simulink model "mult_friction_observer"  (R2021a)
settings: Solver=FixedStepAuto  StartTime=0.0  StopTime=10.0  RelTol=1e-3
model workspace (MAT data in the model file):
  C = [1  0  0  0  0  0  0  0; 0  1  0  0  0  0  0  0; 0  0  1  0  0  0  0  0; 0  0  0  1  0  0  0  0]
  Gamma = [0.005  0  0  0; 0  0.005  0  0; 0  0  0.005  0; 0  0  0  0.005; 0  0  0  0; 0  0  0  0; 0  0  0  0; 0  0  0  0]
  L = [0.86054447364  -0.080292367616  -0.128389264309  0.0921786693579; 0.0643400875833  0.825287721844  0.151017179007  0.010258969185; -0.0245436500305  -0.0437560245931  0.828239855806  -0.0359294386871; -0.0985279277998  0.00654816106119  0.213243264372  0.710326675841; -86.465018388  -7.61905487874  13.7748818427  -3.05301802345; -2.05392908471  -74.8278985038  -8.19625899202  -1.35897353285; 5.97220378745  -11.304802381  -76.7309175474  -0.134671122007; -11.4863013293  -16.7435461743  -5.18969499217  -60.1810056818]
  Phi = [1  0  0  0  -0.0016511627907  0  0  0; 0  1  0  0  0  -0.0016511627907  0  0; 0  0  1  0  0  0  -0.00160888284614  0; 0  0  0  1  0  0  0  -0.00160888284614; 0  0  0  0  1  0  0  0; 0  0  0  0  0  1  0  0; 0  0  0  0  0  0  1  0; 0  0  0  0  0  0  0  1]
  Ts = 0.005
settings Model: OrderedModelArguments=off  Creator=Henrique Mesquita  LastModifiedBy=Henrique Mesquita

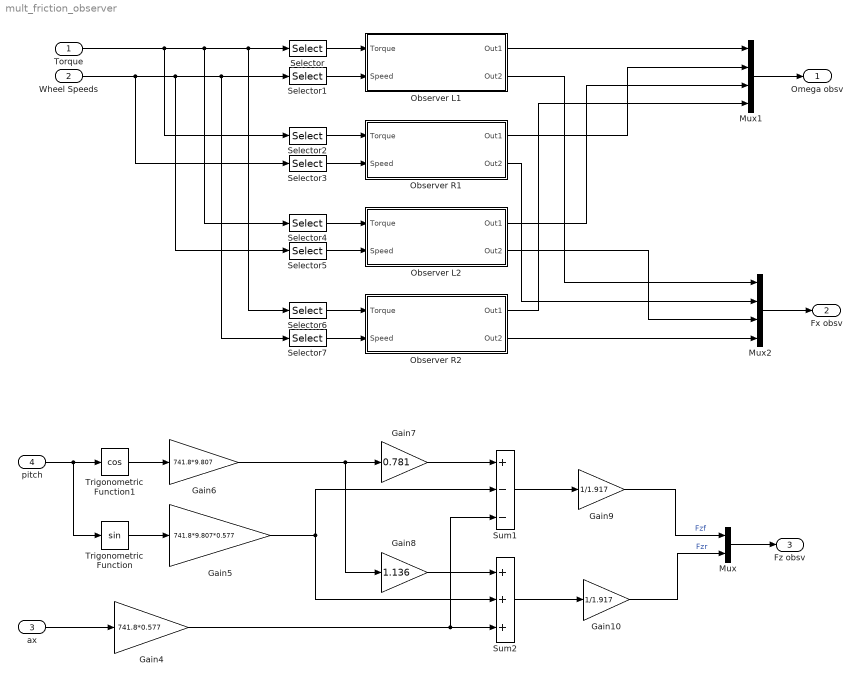
== system mult_friction_observer ==
  Torque : Inport  PortDimensions=4
  Wheel Speeds : Inport  Port=2  PortDimensions=4
  ax : Inport  Port=3
  pitch : Inport  Port=4
  Gain10 : Gain  Gain=1/1.917
  Gain4 : Gain  Gain=741.8*0.577
  Gain5 : Gain  Gain=741.8*9.807*0.577
  Gain6 : Gain  Gain=741.8*9.807
  Gain7 : Gain  Gain=0.781
  Gain8 : Gain  Gain=1.136
  Gain9 : Gain  Gain=1/1.917
  Mux : Mux  Inputs=2
  Mux1 : Mux
  Mux2 : Mux
  Observer L1 : Subsystem
  Observer L2 : Subsystem
  Observer R1 : Subsystem
  Observer R2 : Subsystem
  Selector : Selector  InputPortWidth=4  IndexOptions=Index vector (dialog)  Indices=[1]  OutputSizes=1
  Selector1 : Selector  InputPortWidth=4  IndexOptions=Index vector (dialog)  Indices=[1]  OutputSizes=1
  Selector2 : Selector  InputPortWidth=4  IndexOptions=Index vector (dialog)  Indices=[1]  OutputSizes=1
  Selector3 : Selector  InputPortWidth=4  IndexOptions=Index vector (dialog)  Indices=[2]  OutputSizes=1
  Selector4 : Selector  InputPortWidth=4  IndexOptions=Index vector (dialog)  Indices=[3]  OutputSizes=1
  Selector5 : Selector  InputPortWidth=4  IndexOptions=Index vector (dialog)  Indices=[3]  OutputSizes=1
  Selector6 : Selector  InputPortWidth=4  IndexOptions=Index vector (dialog)  Indices=[4]  OutputSizes=1
  Selector7 : Selector  InputPortWidth=4  IndexOptions=Index vector (dialog)  Indices=[4]  OutputSizes=1
  Sum1 : Sum  Inputs=+--
  Sum2 : Sum  Inputs=+++
  Trigonometric Function : Trigonometry
  Trigonometric Function1 : Trigonometry  Operator=cos
  Omega obsv : Outport
  Fx obsv : Outport  Port=2
  Fz obsv : Outport  Port=3
  wires:
  pitch/1 -> Trigonometric Function/1, Trigonometric Function1/1
  Trigonometric Function/1 -> Gain5/1
  Trigonometric Function1/1 -> Gain6/1
  Gain6/1 -> Gain8/1, Gain7/1
  Gain7/1 -> Sum1/1
  Gain8/1 -> Sum2/1
  Gain5/1 -> Sum2/2, Sum1/2
  ax/1 -> Gain4/1
  Gain4/1 -> Sum1/3, Sum2/3
  Sum1/1 -> Gain9/1
  Sum2/1 -> Gain10/1
  Gain9/1 -> Mux/1  "Fzf"
  Gain10/1 -> Mux/2  "Fzr"
  Mux/1 -> Fz obsv/1
  Wheel Speeds/1 -> Selector3/1, Selector5/1, Selector7/1, Selector1/1
  Torque/1 -> Selector2/1, Selector6/1, Selector/1, Selector4/1
  Selector/1 -> Observer L1/1(Torque)
  Selector1/1 -> Observer L1/2(Speed)
  Selector2/1 -> Observer R1/1(Torque)
  Selector3/1 -> Observer R1/2(Speed)
  Selector4/1 -> Observer L2/1(Torque)
  Selector5/1 -> Observer L2/2(Speed)
  Selector6/1 -> Observer R2/1(Torque)
  Selector7/1 -> Observer R2/2(Speed)
  Observer L1/1(Out1) -> Mux1/1
  Observer R1/1(Out1) -> Mux1/2
  Observer L2/1(Out1) -> Mux1/3
  Observer R2/1(Out1) -> Mux1/4
  Observer L1/2(Out2) -> Mux2/1
  Observer R1/2(Out2) -> Mux2/2
  Observer L2/2(Out2) -> Mux2/3
  Observer R2/2(Out2) -> Mux2/4
  Mux2/1 -> Fx obsv/1
  Mux1/1 -> Omega obsv/1

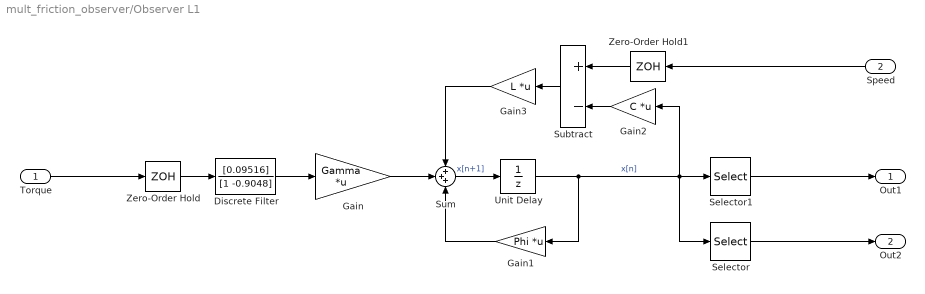
== system mult_friction_observer/Observer L1 ==
  Torque : Inport
  Speed : Inport  Port=2
  Discrete Filter : DiscreteFilter  Numerator=[0.09516]  Denominator=[1 -0.9048]
  Gain : Gain  Gain=Gamma  Multiplication=Matrix(K*u)
  Gain1 : Gain  Gain=Phi  Multiplication=Matrix(K*u)
  Gain2 : Gain  Gain=C  Multiplication=Matrix(K*u)
  Gain3 : Gain  Gain=L  Multiplication=Matrix(K*u)
  Selector : Selector  InputPortWidth=8  IndexOptions=Index vector (dialog)  Indices=[5 6 7 8]  OutputSizes=1
  Selector1 : Selector  InputPortWidth=8  IndexOptions=Index vector (dialog)  Indices=[1 2 3 4]  OutputSizes=1
  Subtract : Sum  Inputs=+-
  Sum : Sum  Inputs=+++
  Unit Delay : UnitDelay  SampleTime=Ts  HasFrameUpgradeWarning=on
  Zero-Order Hold : ZeroOrderHold  SampleTime=Ts
  Zero-Order Hold1 : ZeroOrderHold  SampleTime=Ts
  Out1 : Outport
  Out2 : Outport  Port=2
  wires:
  Sum/1 -> Unit Delay/1  "x[n+1]"
  Unit Delay/1 -> Selector1/1, Selector/1, Gain2/1, Gain1/1  "x[n]"
  Gain3/1 -> Sum/1
  Zero-Order Hold/1 -> Discrete Filter/1
  Subtract/1 -> Gain3/1
  Gain2/1 -> Subtract/2
  Gain1/1 -> Sum/3
  Gain/1 -> Sum/2
  Zero-Order Hold1/1 -> Subtract/1
  Discrete Filter/1 -> Gain/1
  Selector/1 -> Out2/1
  Torque/1 -> Zero-Order Hold/1
  Speed/1 -> Zero-Order Hold1/1
  Selector1/1 -> Out1/1

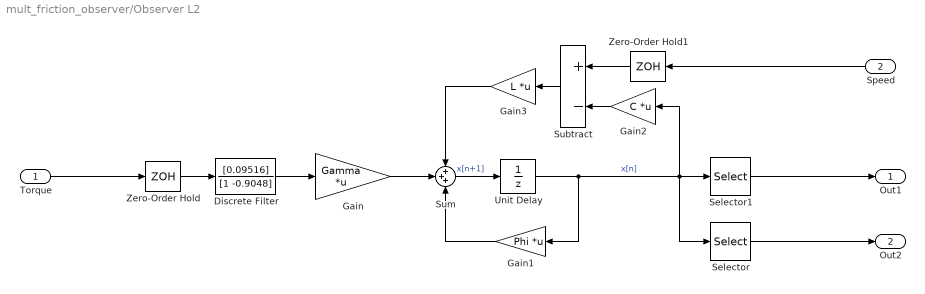
== system mult_friction_observer/Observer L2 ==
  Torque : Inport
  Speed : Inport  Port=2
  Discrete Filter : DiscreteFilter  Numerator=[0.09516]  Denominator=[1 -0.9048]
  Gain : Gain  Gain=Gamma  Multiplication=Matrix(K*u)
  Gain1 : Gain  Gain=Phi  Multiplication=Matrix(K*u)
  Gain2 : Gain  Gain=C  Multiplication=Matrix(K*u)
  Gain3 : Gain  Gain=L  Multiplication=Matrix(K*u)
  Selector : Selector  InputPortWidth=8  IndexOptions=Index vector (dialog)  Indices=[5 6 7 8]  OutputSizes=1
  Selector1 : Selector  InputPortWidth=8  IndexOptions=Index vector (dialog)  Indices=[1 2 3 4]  OutputSizes=1
  Subtract : Sum  Inputs=+-
  Sum : Sum  Inputs=+++
  Unit Delay : UnitDelay  SampleTime=Ts  HasFrameUpgradeWarning=on
  Zero-Order Hold : ZeroOrderHold  SampleTime=Ts
  Zero-Order Hold1 : ZeroOrderHold  SampleTime=Ts
  Out1 : Outport
  Out2 : Outport  Port=2
  wires:
  Sum/1 -> Unit Delay/1  "x[n+1]"
  Unit Delay/1 -> Selector1/1, Selector/1, Gain2/1, Gain1/1  "x[n]"
  Gain3/1 -> Sum/1
  Zero-Order Hold/1 -> Discrete Filter/1
  Subtract/1 -> Gain3/1
  Gain2/1 -> Subtract/2
  Gain1/1 -> Sum/3
  Gain/1 -> Sum/2
  Zero-Order Hold1/1 -> Subtract/1
  Discrete Filter/1 -> Gain/1
  Selector/1 -> Out2/1
  Torque/1 -> Zero-Order Hold/1
  Speed/1 -> Zero-Order Hold1/1
  Selector1/1 -> Out1/1

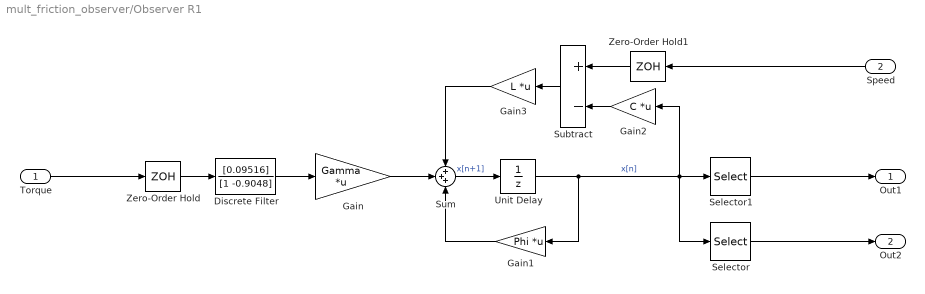
== system mult_friction_observer/Observer R1 ==
  Torque : Inport
  Speed : Inport  Port=2
  Discrete Filter : DiscreteFilter  Numerator=[0.09516]  Denominator=[1 -0.9048]
  Gain : Gain  Gain=Gamma  Multiplication=Matrix(K*u)
  Gain1 : Gain  Gain=Phi  Multiplication=Matrix(K*u)
  Gain2 : Gain  Gain=C  Multiplication=Matrix(K*u)
  Gain3 : Gain  Gain=L  Multiplication=Matrix(K*u)
  Selector : Selector  InputPortWidth=8  IndexOptions=Index vector (dialog)  Indices=[5 6 7 8]  OutputSizes=1
  Selector1 : Selector  InputPortWidth=8  IndexOptions=Index vector (dialog)  Indices=[1 2 3 4]  OutputSizes=1
  Subtract : Sum  Inputs=+-
  Sum : Sum  Inputs=+++
  Unit Delay : UnitDelay  SampleTime=Ts  HasFrameUpgradeWarning=on
  Zero-Order Hold : ZeroOrderHold  SampleTime=Ts
  Zero-Order Hold1 : ZeroOrderHold  SampleTime=Ts
  Out1 : Outport
  Out2 : Outport  Port=2
  wires:
  Sum/1 -> Unit Delay/1  "x[n+1]"
  Unit Delay/1 -> Selector1/1, Selector/1, Gain2/1, Gain1/1  "x[n]"
  Gain3/1 -> Sum/1
  Zero-Order Hold/1 -> Discrete Filter/1
  Subtract/1 -> Gain3/1
  Gain2/1 -> Subtract/2
  Gain1/1 -> Sum/3
  Gain/1 -> Sum/2
  Zero-Order Hold1/1 -> Subtract/1
  Discrete Filter/1 -> Gain/1
  Selector/1 -> Out2/1
  Torque/1 -> Zero-Order Hold/1
  Speed/1 -> Zero-Order Hold1/1
  Selector1/1 -> Out1/1

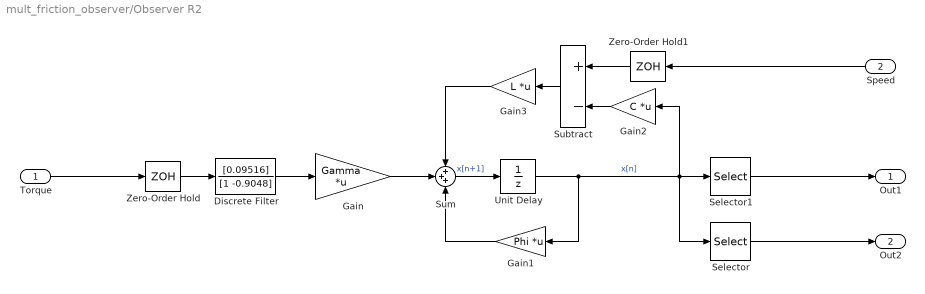
== system mult_friction_observer/Observer R2 ==
  Torque : Inport
  Speed : Inport  Port=2
  Discrete Filter : DiscreteFilter  Numerator=[0.09516]  Denominator=[1 -0.9048]
  Gain : Gain  Gain=Gamma  Multiplication=Matrix(K*u)
  Gain1 : Gain  Gain=Phi  Multiplication=Matrix(K*u)
  Gain2 : Gain  Gain=C  Multiplication=Matrix(K*u)
  Gain3 : Gain  Gain=L  Multiplication=Matrix(K*u)
  Selector : Selector  InputPortWidth=8  IndexOptions=Index vector (dialog)  Indices=[5 6 7 8]  OutputSizes=1
  Selector1 : Selector  InputPortWidth=8  IndexOptions=Index vector (dialog)  Indices=[1 2 3 4]  OutputSizes=1
  Subtract : Sum  Inputs=+-
  Sum : Sum  Inputs=+++
  Unit Delay : UnitDelay  SampleTime=Ts  HasFrameUpgradeWarning=on
  Zero-Order Hold : ZeroOrderHold  SampleTime=Ts
  Zero-Order Hold1 : ZeroOrderHold  SampleTime=Ts
  Out1 : Outport
  Out2 : Outport  Port=2
  wires:
  Sum/1 -> Unit Delay/1  "x[n+1]"
  Unit Delay/1 -> Selector1/1, Selector/1, Gain2/1, Gain1/1  "x[n]"
  Gain3/1 -> Sum/1
  Zero-Order Hold/1 -> Discrete Filter/1
  Subtract/1 -> Gain3/1
  Gain2/1 -> Subtract/2
  Gain1/1 -> Sum/3
  Gain/1 -> Sum/2
  Zero-Order Hold1/1 -> Subtract/1
  Discrete Filter/1 -> Gain/1
  Selector/1 -> Out2/1
  Torque/1 -> Zero-Order Hold/1
  Speed/1 -> Zero-Order Hold1/1
  Selector1/1 -> Out1/1
